simulink model "dev_switch_ekf"  (Simulink 7.0)
settings: Solver=FixedStepDiscrete  StartTime=0  StopTime=100  FixedStep=1e-3  RelTol=1e-3
undefined symbols (not defined in the file): l_fts, Q_in, R_n9, ts, zmsr
libraries: simulink x14, DLRwalkerLib x3, DLRHumanoid x2
(part 1 of 2)
settings Model: Creator=raje_ra  LastModifiedBy=raje_ra  ExtModeAutoUpdateStatusClock=off

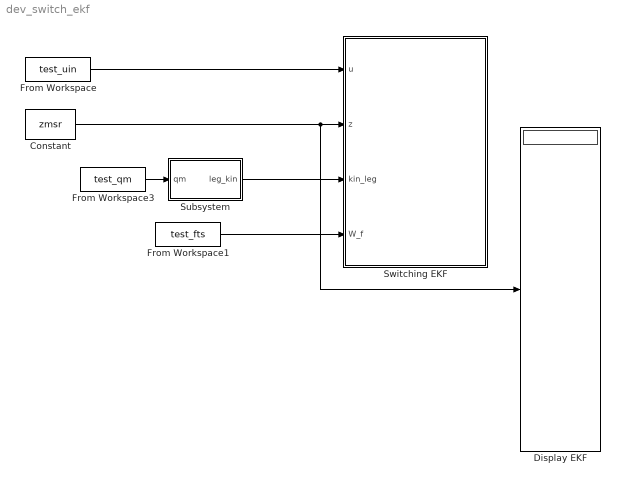
== system dev_switch_ekf ==
  Constant : Constant  Value=zmsr  OutDataType=sfix(16)  OutScaling=2^0
  Display EKF : Display
  From Workspace : FromWorkspace  VariableName=test_uin  SampleTime=0  OutputAfterFinalValue=Setting to zero
  From Workspace1 : FromWorkspace  VariableName=test_fts  SampleTime=0  OutputAfterFinalValue=Setting to zero
  From Workspace3 : FromWorkspace  VariableName=test_qm  SampleTime=0  OutputAfterFinalValue=Setting to zero
  Subsystem : Subsystem
  Switching EKF : Subsystem
  wires:
  From Workspace3/1 -> Subsystem/1(qm)
  Subsystem/1(leg_kin) -> Switching EKF/3(kin_leg)
  From Workspace1/1 -> Switching EKF/4(W_f)
  From Workspace/1 -> Switching EKF/1(u)
  Constant/1 -> Switching EKF/2(z), Display EKF/1

== system dev_switch_ekf/Subsystem ==
  qm : Inport  OutDataType=sfix(16)  OutScaling=2^0
  Bus Creator : BusCreator
  Fkin_leg_l : DLRHumanoid/Fkin_leg_l  SystemSampleTime=-1
  Fkin_leg_r : DLRHumanoid/Fkin_leg_r  SystemSampleTime=-1
  J_leg_l : Subsystem  AncestorBlock=DLRHumanoid/J_leg_l
  J_leg_r : Subsystem  AncestorBlock=DLRHumanoid/J_leg_r
  leg_kin : Outport  OutDataType=sfix(16)  OutScaling=2^0
  wires:
  qm/1 -> Fkin_leg_r/1, Fkin_leg_l/1, J_leg_r/1(q), J_leg_l/1(q)
  Fkin_leg_r/1 -> Bus Creator/1  "Fkin_leg_r"
  Bus Creator/1 -> leg_kin/1
  Fkin_leg_l/1 -> Bus Creator/2  "Fkin_leg_l"
  J_leg_r/1(J) -> Bus Creator/3  "J_leg_r"
  J_leg_l/1(J) -> Bus Creator/4  "J_leg_l"

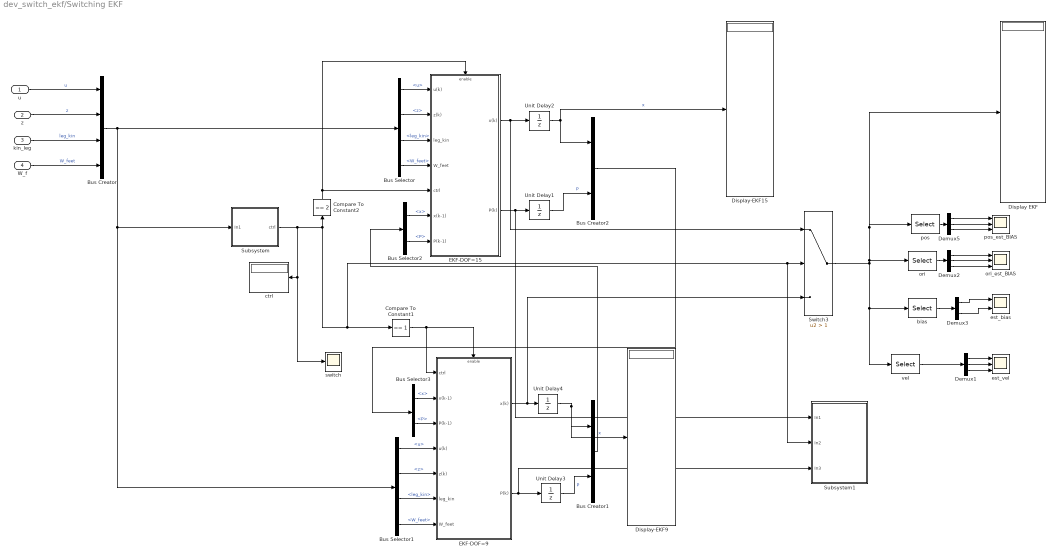
== system dev_switch_ekf/Switching EKF ==
  u : Inport
  z : Inport  Port=2
  kin_leg : Inport  Port=3
  W_f : Inport  Port=4
  Bus Creator : BusCreator
  Bus Creator1 : BusCreator  Inputs=2
  Bus Creator2 : BusCreator  Inputs=2
  Bus Selector : BusSelector  OutputSignals=u,z,leg_kin,W_feet
  Bus Selector1 : BusSelector  OutputSignals=u,z,leg_kin,W_feet
  Bus Selector2 : BusSelector  OutputSignals=x,P
  Bus Selector3 : BusSelector  OutputSignals=x,P
  Compare To Constant1 : simulink/Logic and Bit Operations/Compare To Constant  SystemSampleTime=-1  relop===  const=1  LogicOutDataTypeMode=uint8  ZeroCross=off
  Compare To Constant2 : simulink/Logic and Bit Operations/Compare To Constant  Orientation=up  SystemSampleTime=-1  relop===  const=2  LogicOutDataTypeMode=uint8  ZeroCross=off
  Demux1 : Demux  Outputs=3
  Demux2 : Demux  Outputs=3
  Demux3 : Demux  Outputs=2
  Demux5 : Demux  Outputs=3
  Display EKF : Display
  Display-EKF15 : Display
  Display-EKF9 : Display
  EKF-DOF=15 : Subsystem
  EKF-DOF=9 : Subsystem
  Subsystem : Subsystem
  Subsystem1 : Subsystem
  Switch3 : Switch  Criteria=u2 > Threshold  Threshold=1  OutDataType=sfix(16)  OutScaling=2^0
  Unit Delay1 : UnitDelay  X0=zeros(15)  SampleTime=-1
  Unit Delay2 : UnitDelay  X0=zeros(15,1)  SampleTime=-1
  Unit Delay3 : UnitDelay  X0=eye(15)  SampleTime=-1
  Unit Delay4 : UnitDelay  X0=zeros(15,1)  SampleTime=-1
  bias : Selector  InputPortWidth=15  IndexOptions=Index vector (dialog)  Indices=10:15  OutputSizes=1
  ctrl : Display
      settings: Decimation=100
  est_bias : Scope  NumInputPorts=2
      settings: TickLabels=on  TimeRange=10  YMin=-0.08~-0.14  YMax=0.14~0.06  SaveName=ScopeData117
  est_vel : Scope  NumInputPorts=3
      settings: TickLabels=on  TimeRange=1  YMin=-0.025~-8.67362e-19~-0.02  YMax=0.0025~0.04~0.002
  ori : Selector  InputPortWidth=15  IndexOptions=Index vector (dialog)  Indices=4:6  OutputSizes=1
  ori_est_BIAS : Scope  NumInputPorts=3
      settings: TickLabels=on  TimeRange=10  YMin=-0.009000000000000001~-0.12~-0.026  YMax=-0.003000000000000001~0.04000000000000001~-0.012  SaveName=ScopeData109
  pos : Selector  InputPortWidth=15  IndexOptions=Index vector (dialog)  Indices=1:3  OutputSizes=1
  pos_est_BIAS : Scope  NumInputPorts=3
      settings: TickLabels=on  TimeRange=30  YMin=-0.004~-0.025~1.161  YMax=0.0055~0.275~1.175  SaveName=ScopeData128
  switch : Scope
      settings: TickLabels=on  TimeRange=1  YMin=-0.025  YMax=0.0025  SaveName=ScopeData4
  vel : Selector  InputPortWidth=15  IndexOptions=Index vector (dialog)  Indices=7:9  OutputSizes=1
  wires:
  ori/1 -> Demux2/1
  Demux2/1 -> ori_est_BIAS/1
  Demux2/2 -> ori_est_BIAS/2
  Demux2/3 -> ori_est_BIAS/3
  bias/1 -> Demux3/1
  Demux3/1 -> est_bias/1
  Demux3/2 -> est_bias/2
  pos/1 -> Demux5/1
  Demux5/1 -> pos_est_BIAS/1
  Demux5/2 -> pos_est_BIAS/2
  Demux5/3 -> pos_est_BIAS/3
  u/1 -> Bus Creator/1  "u"
  z/1 -> Bus Creator/2  "z"
  kin_leg/1 -> Bus Creator/3  "leg_kin"
  W_f/1 -> Bus Creator/4  "W_feet"
  Bus Creator/1 -> Bus Selector/1, Bus Selector1/1, Subsystem/1(In1)
  Bus Selector/1 -> EKF-DOF=15/1(u(k))  "<u>"
  Bus Selector/2 -> EKF-DOF=15/2(z(k))  "<z>"
  Bus Selector/3 -> EKF-DOF=15/3(leg_kin)  "<leg_kin>"
  Bus Selector/4 -> EKF-DOF=15/4(W_feet)  "<W_feet>"
  Bus Selector1/1 -> EKF-DOF=9/4(u(k))  "<u>"
  Bus Selector1/2 -> EKF-DOF=9/5(z(k))  "<z>"
  Bus Selector1/3 -> EKF-DOF=9/6(leg_kin)  "<leg_kin>"
  Bus Selector1/4 -> EKF-DOF=9/7(W_feet)  "<W_feet>"
  EKF-DOF=15/1(x(k)) -> Unit Delay2/1, Switch3/1
  EKF-DOF=15/2(P(k)) -> Unit Delay1/1, Subsystem1/1(In1)
  Compare To Constant1/1 -> EKF-DOF=9/1(ctrl), EKF-DOF=9/Enable
  Subsystem/1(ctrl) -> Compare To Constant1/1, Switch3/2, Subsystem1/2(In2), Compare To Constant2/1, ctrl/1, switch/1
  EKF-DOF=9/1(x(k)) -> Unit Delay4/1, Switch3/3
  EKF-DOF=9/2(P(k)) -> Unit Delay3/1, Subsystem1/3(In3)
  Unit Delay4/1 -> Bus Creator1/1, Display-EKF9/1  "x"
  Unit Delay3/1 -> Bus Creator1/2  "P"
  Unit Delay2/1 -> Bus Creator2/1, Display-EKF15/1  "x"
  Unit Delay1/1 -> Bus Creator2/2  "P"
  Bus Selector2/1 -> EKF-DOF=15/6(x(k-1))  "<x>"
  Bus Selector2/2 -> EKF-DOF=15/7(P(k-1))  "<P>"
  Bus Selector3/1 -> EKF-DOF=9/2(x(k-1))  "<x>"
  Bus Selector3/2 -> EKF-DOF=9/3(P(k-1))  "<P>"
  Bus Creator2/1 -> Bus Selector3/1
  Bus Creator1/1 -> Bus Selector2/1
  Switch3/1 -> ori/1, pos/1, Display EKF/1, bias/1, vel/1
  Compare To Constant2/1 -> EKF-DOF=15/5(ctrl), EKF-DOF=15/Enable
  Demux1/1 -> est_vel/1
  Demux1/2 -> est_vel/2
  Demux1/3 -> est_vel/3
  vel/1 -> Demux1/1

== system dev_switch_ekf/Subsystem/J_leg_l ==
  q : Inport
  Reshape10 : Reshape  OutputDimensionality=Customize  OutputDimensions=[6,6]
  S-Function1 : S-Function  FunctionName=sJ_leg_l  Parameters=kinpar
  J : Outport
  wires:
  q/1 -> S-Function1/1
  Reshape10/1 -> J/1
  S-Function1/1 -> Reshape10/1

== system dev_switch_ekf/Subsystem/J_leg_r ==
  q : Inport
  Reshape10 : Reshape  OutputDimensionality=Customize  OutputDimensions=[6,6]
  S-Function4 : S-Function  FunctionName=sJ_leg_r  Parameters=kinpar
  J : Outport
  wires:
  S-Function4/1 -> Reshape10/1
  Reshape10/1 -> J/1
  q/1 -> S-Function4/1

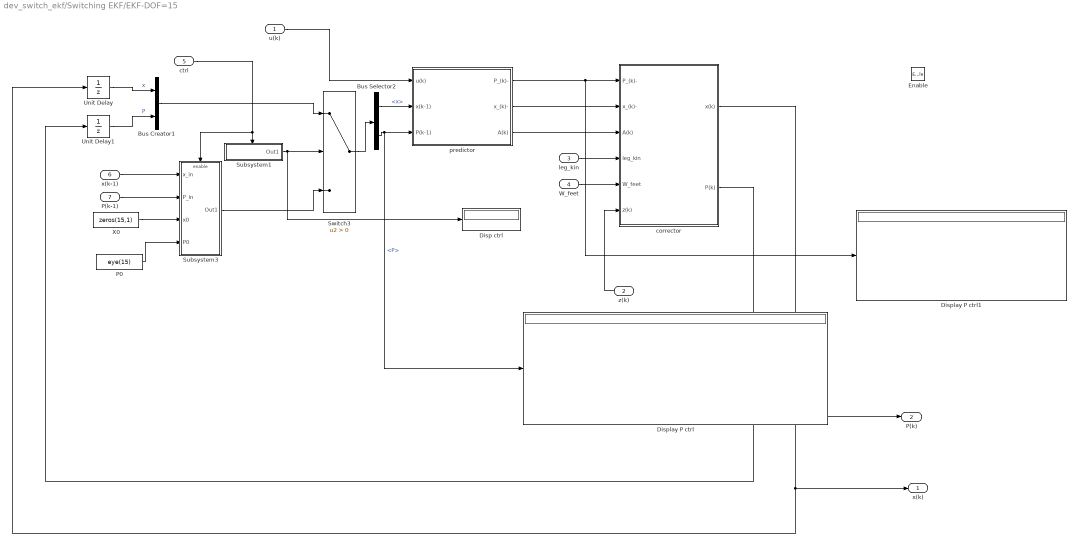
== system dev_switch_ekf/Switching EKF/EKF-DOF=15 ==
  u(k) : Inport  OutDataType=sfix(16)  OutScaling=2^0
  z(k) : Inport  Orientation=left  Port=2  OutDataType=sfix(16)  OutScaling=2^0
  leg_kin : Inport  Port=3  OutDataType=sfix(16)  OutScaling=2^0
  W_feet : Inport  Port=4  OutDataType=sfix(16)  OutScaling=2^0
  ctrl : Inport  Port=5  OutDataType=sfix(16)  OutScaling=2^0
  x(k-1) : Inport  Port=6  OutDataType=sfix(16)  OutScaling=2^0
  P(k-1) : Inport  Port=7  OutDataType=sfix(16)  OutScaling=2^0
  Enable : EnablePort  StatesWhenEnabling=reset
  Bus Creator1 : BusCreator  Inputs=2
  Bus Selector2 : BusSelector  OutputSignals=x,P
  Disp ctrl : Display
  Display P ctrl : Display
  Display P ctrl1 : Display
  P0 : Constant  Value=eye(15)  VectorParams1D=off  OutDataType=sfix(16)  OutScaling=2^0
  Subsystem1 : Subsystem
  Subsystem3 : Subsystem
  Switch3 : Switch  Criteria=u2 > Threshold  OutDataType=sfix(16)  OutScaling=2^0
  Unit Delay : UnitDelay  X0=zeros(15,1)  SampleTime=ts
  Unit Delay1 : UnitDelay  X0=zeros(15)  SampleTime=ts
  X0 : Constant  Value=zeros(15,1)  OutDataType=sfix(16)  OutScaling=2^0
  corrector : Subsystem
  predictor : Subsystem
  x(k) : Outport  OutDataType=sfix(16)  OutScaling=2^0
  P(k) : Outport  Port=2  OutDataType=sfix(16)  OutScaling=2^0
  wires:
  corrector/2(P(k)) -> Unit Delay1/1, P(k)/1
  predictor/1(P_(k)-) -> corrector/1(P_(k)-), Display P ctrl1/1
  corrector/1(x(k)) -> Unit Delay/1, x(k)/1
  predictor/2(x_(k)-) -> corrector/2(x_(k)-)
  u(k)/1 -> predictor/1(u(k))
  leg_kin/1 -> corrector/4(leg_kin)
  W_feet/1 -> corrector/5(W_feet)
  z(k)/1 -> corrector/6(z(k))
  predictor/3(A(k)) -> corrector/3(A(k))
  Subsystem1/1(Out1) -> Switch3/2, Disp ctrl/1
  ctrl/1 -> Subsystem1/Enable, Subsystem3/Enable
  Subsystem3/1(Out1) -> Switch3/3
  X0/1 -> Subsystem3/3(x0)
  P0/1 -> Subsystem3/4(P0)
  x(k-1)/1 -> Subsystem3/1(x_in)
  P(k-1)/1 -> Subsystem3/2(P_in)
  Unit Delay/1 -> Bus Creator1/1  "x"
  Unit Delay1/1 -> Bus Creator1/2  "P"
  Bus Creator1/1 -> Switch3/1
  Switch3/1 -> Bus Selector2/1
  Bus Selector2/1 -> predictor/2(x(k-1))  "<x>"
  Bus Selector2/2 -> predictor/3(P(k-1)), Display P ctrl/1  "<P>"

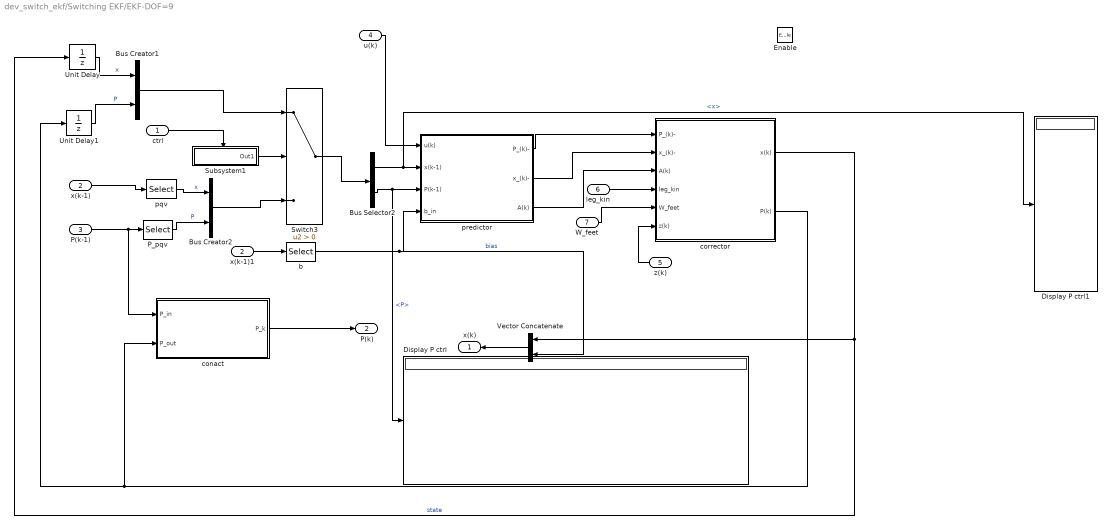
== system dev_switch_ekf/Switching EKF/EKF-DOF=9 ==
  ctrl : Inport  OutDataType=sfix(16)  OutScaling=2^0
  x(k-1) : Inport  Port=2  OutDataType=sfix(16)  OutScaling=2^0
  P(k-1) : Inport  Port=3  OutDataType=sfix(16)  OutScaling=2^0
  u(k) : Inport  Port=4  OutDataType=sfix(16)  OutScaling=2^0
  z(k) : Inport  Orientation=left  Port=5  OutDataType=sfix(16)  OutScaling=2^0
  leg_kin : Inport  Port=6  OutDataType=sfix(16)  OutScaling=2^0
  W_feet : Inport  Port=7  OutDataType=sfix(16)  OutScaling=2^0
  Enable : EnablePort  StatesWhenEnabling=reset
  Bus Creator1 : BusCreator  Inputs=2
  Bus Creator2 : BusCreator  Inputs=2
  Bus Selector2 : BusSelector  OutputSignals=x,P
  Display P ctrl : Display
  Display P ctrl1 : Display
  P_pqv : Selector  NumberOfDimensions=2  InputPortWidth=15  IndexOptions=Index vector (dialog),Index vector (dialog)  Indices=1:9,1:9  OutputSizes=1,1
  Subsystem1 : Subsystem
  Switch3 : Switch  Criteria=u2 > Threshold  OutDataType=sfix(16)  OutScaling=2^0
  Unit Delay : UnitDelay  X0=zeros(9,1)  SampleTime=ts
  Unit Delay1 : UnitDelay  X0=eye(9)  SampleTime=ts
  Vector Concatenate : Concatenate  Orientation=left  Mode=Vector
  b : Selector  InputPortWidth=15  IndexOptions=Index vector (dialog)  Indices=10:15  OutputSizes=1
  conact : Stateflow chart
  corrector : Subsystem
  pqv : Selector  InputPortWidth=15  IndexOptions=Index vector (dialog)  Indices=1:9  OutputSizes=1
  predictor : Subsystem
  x(k-1)1 : InportShadow  Port=2  OutDataType=sfix(16)  OutScaling=2^0  LatchByCopyingInsideSignal=off
  x(k) : Outport  Orientation=left  OutDataType=sfix(16)  OutScaling=2^0
  P(k) : Outport  Port=2  OutDataType=sfix(16)  OutScaling=2^0
  wires:
  predictor/3(A(k)) -> corrector/3(A(k))
  z(k)/1 -> corrector/6(z(k))
  W_feet/1 -> corrector/5(W_feet)
  leg_kin/1 -> corrector/4(leg_kin)
  u(k)/1 -> predictor/1(u(k))
  predictor/2(x_(k)-) -> corrector/2(x_(k)-)
  corrector/1(x(k)) -> Vector Concatenate/1, Unit Delay/1  "state"
  predictor/1(P_(k)-) -> corrector/1(P_(k)-)
  corrector/2(P(k)) -> Unit Delay1/1, conact/2(P_out)
  Subsystem1/1(Out1) -> Switch3/2
  x(k-1)/1 -> pqv/1
  ctrl/1 -> Subsystem1/Enable
  P(k-1)/1 -> P_pqv/1, conact/1(P_in)
  b/1 -> predictor/4(b_in), Vector Concatenate/2  "bias"
  Vector Concatenate/1 -> x(k)/1
  conact/1(P_k) -> P(k)/1
  Unit Delay/1 -> Bus Creator1/1  "x"
  Unit Delay1/1 -> Bus Creator1/2  "P"
  Bus Creator1/1 -> Switch3/1
  P_pqv/1 -> Bus Creator2/2  "P"
  pqv/1 -> Bus Creator2/1  "x"
  Bus Creator2/1 -> Switch3/3
  Switch3/1 -> Bus Selector2/1
  Bus Selector2/1 -> predictor/2(x(k-1)), Display P ctrl1/1  "<x>"
  Bus Selector2/2 -> predictor/3(P(k-1)), Display P ctrl/1  "<P>"
  x(k-1)1/1 -> b/1

== system dev_switch_ekf/Switching EKF/Subsystem ==
  note: 1..single left leg
      | 2.. single right leg
      | 3.. double support
      | 4.. flying
  In1 : Inport
  Bus Selector2 : BusSelector  OutputSignals=W_feet
  Demux : Demux  Outputs=2
  ZMP Calculator : Subsystem
  conact : Stateflow chart
  ctrl : Outport
  wires:
  Bus Selector2/1 -> Demux/1  "<W_feet>"
  Demux/2 -> ZMP Calculator/2(WL)
  Demux/1 -> ZMP Calculator/1(WR)
  ZMP Calculator/1(pcalc) -> conact/1(zmp)
  ZMP Calculator/2(cnt_state) -> conact/2(state)
  In1/1 -> Bus Selector2/1
  conact/1(y) -> ctrl/1

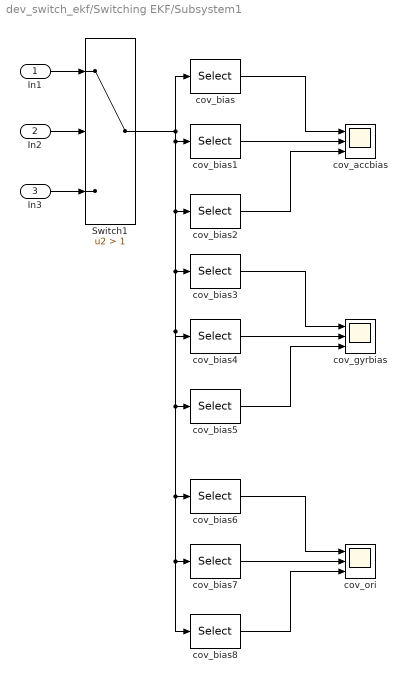
== system dev_switch_ekf/Switching EKF/Subsystem1 ==
  In1 : Inport
  In2 : Inport  Port=2
  In3 : Inport  Port=3
  Switch1 : Switch  Criteria=u2 > Threshold  Threshold=1  OutDataType=sfix(16)  OutScaling=2^0
  cov_accbias : Scope  NumInputPorts=3
      settings: TickLabels=on  TimeRange=1  YMin=-0.025~-8.67362e-19~-0.02  YMax=0.0025~0.04~0.002
  cov_bias : Selector  NumberOfDimensions=2  InputPortWidth=15  IndexOptions=Index vector (dialog),Index vector (dialog)  Indices=10,10  OutputSizes=1,1
  cov_bias1 : Selector  NumberOfDimensions=2  InputPortWidth=15  IndexOptions=Index vector (dialog),Index vector (dialog)  Indices=11,11  OutputSizes=1,1
  cov_bias2 : Selector  NumberOfDimensions=2  InputPortWidth=15  IndexOptions=Index vector (dialog),Index vector (dialog)  Indices=12,12  OutputSizes=1,1
  cov_bias3 : Selector  NumberOfDimensions=2  InputPortWidth=15  IndexOptions=Index vector (dialog),Index vector (dialog)  Indices=13,13  OutputSizes=1,1
  cov_bias4 : Selector  NumberOfDimensions=2  InputPortWidth=15  IndexOptions=Index vector (dialog),Index vector (dialog)  Indices=14,14  OutputSizes=1,1
  cov_bias5 : Selector  NumberOfDimensions=2  InputPortWidth=15  IndexOptions=Index vector (dialog),Index vector (dialog)  Indices=15,15  OutputSizes=1,1
  cov_bias6 : Selector  NumberOfDimensions=2  InputPortWidth=15  IndexOptions=Index vector (dialog),Index vector (dialog)  Indices=4,4  OutputSizes=1,1
  cov_bias7 : Selector  NumberOfDimensions=2  InputPortWidth=15  IndexOptions=Index vector (dialog),Index vector (dialog)  Indices=5,5  OutputSizes=1,1
  cov_bias8 : Selector  NumberOfDimensions=2  InputPortWidth=15  IndexOptions=Index vector (dialog),Index vector (dialog)  Indices=6,6  OutputSizes=1,1
  cov_gyrbias : Scope  NumInputPorts=3
      settings: TickLabels=on  TimeRange=1  YMin=-0.025~-8.67362e-19~-0.02  YMax=0.0025~0.04~0.002  SaveName=ScopeData2
  cov_ori : Scope  NumInputPorts=3
      settings: TickLabels=on  TimeRange=10  YMin=4e-12~0~4e-12  YMax=1.4e-11~7.000000000000001e-09~1.8e-11  SaveName=ScopeData3
  wires:
  Switch1/1 -> cov_bias/1, cov_bias1/1, cov_bias2/1, cov_bias3/1, cov_bias4/1, cov_bias5/1, cov_bias6/1, cov_bias7/1, cov_bias8/1
  cov_bias/1 -> cov_accbias/1
  cov_bias1/1 -> cov_accbias/2
  cov_bias2/1 -> cov_accbias/3
  cov_bias3/1 -> cov_gyrbias/1
  cov_bias4/1 -> cov_gyrbias/2
  cov_bias5/1 -> cov_gyrbias/3
  In1/1 -> Switch1/1
  In2/1 -> Switch1/2
  In3/1 -> Switch1/3
  cov_bias6/1 -> cov_ori/1
  cov_bias7/1 -> cov_ori/2
  cov_bias8/1 -> cov_ori/3

== system dev_switch_ekf/Switching EKF/EKF-DOF=15/Subsystem1 ==
  Enable : EnablePort  StatesWhenEnabling=reset
  Init/Run  Logik : DLRwalkerLib/Misc/Init//Run  Logik  SystemSampleTime=-1
  Terminator : Terminator
  Out1 : Outport
  wires:
  Init/Run  Logik/1 -> Terminator/1
  Init/Run  Logik/2 -> Out1/1

== system dev_switch_ekf/Switching EKF/EKF-DOF=15/Subsystem3 ==
  x_in : Inport  OutDataType=sfix(16)  OutScaling=2^0
  P_in : Inport  Port=2  OutDataType=sfix(16)  OutScaling=2^0
  x0 : Inport  Port=3  OutDataType=sfix(16)  OutScaling=2^0
  P0 : Inport  Port=4  OutDataType=sfix(16)  OutScaling=2^0
  Enable : EnablePort  ShowOutputPort=on
  Bus Creator1 : BusCreator  Inputs=2
  Bus Creator2 : BusCreator  Inputs=2
  Init/Run  Logik : DLRwalkerLib/Misc/Init//Run  Logik  SystemSampleTime=-1
  Switch : Switch  Criteria=u2 > Threshold  OutDataType=sfix(16)  OutScaling=2^0
  Terminator : Terminator
  Out1 : Outport
  wires:
  Init/Run  Logik/2 -> Switch/2
  Init/Run  Logik/1 -> Terminator/1
  Switch/1 -> Out1/1
  x0/1 -> Bus Creator1/1  "x"
  P0/1 -> Bus Creator1/2  "P"
  Bus Creator1/1 -> Switch/3
  x_in/1 -> Bus Creator2/1  "x"
  P_in/1 -> Bus Creator2/2  "P"
  Bus Creator2/1 -> Switch/1

== system dev_switch_ekf/Switching EKF/EKF-DOF=15/corrector ==
  P_(k)- : Inport  OutDataType=sfix(16)  OutScaling=2^0
  x_(k)- : Inport  Port=2  OutDataType=sfix(16)  OutScaling=2^0
  A(k) : Inport  Port=3  OutDataType=sfix(16)  OutScaling=2^0
  leg_kin : Inport  Port=4  OutDataType=sfix(16)  OutScaling=2^0
  W_feet : Inport  Port=5  OutDataType=sfix(16)  OutScaling=2^0
  z(k) : Inport  Port=6  OutDataType=sfix(16)  OutScaling=2^0
  Bus Selector3 : BusSelector  OutputSignals=Fkin_leg_r,Fkin_leg_l
  Constant : Constant  Value=R_n9  OutDataType=sfix(16)  OutScaling=2^0
  Demux : Demux  Outputs=2
  Eul Rotation : Stateflow chart
  Measurement update1 : Stateflow chart
  Selector1 : Selector  InputPortWidth=15  IndexOptions=Index vector (dialog)  Indices=[1:6]  OutputSizes=1
  ZMP Calculator : Subsystem
  x(k) : Outport  OutDataType=sfix(16)  OutScaling=2^0
  P(k) : Outport  Port=2  OutDataType=sfix(16)  OutScaling=2^0
  wires:
  Measurement update1/1(x_k) -> x(k)/1
  x_(k)-/1 -> Measurement update1/1(x_in), Selector1/1
  Selector1/1 -> Eul Rotation/1(o)
  Eul Rotation/1(g) -> Measurement update1/3(g_in)
  Eul Rotation/2(dg) -> Measurement update1/4(dg_in)
  leg_kin/1 -> Bus Selector3/1
  Bus Selector3/1 -> Measurement update1/5(kin_rf)  "<Fkin_leg_r>"
  Bus Selector3/2 -> Measurement update1/6(kin_lf)  "<Fkin_leg_l>"
  Demux/1 -> ZMP Calculator/2(WR)
  Demux/2 -> ZMP Calculator/1(WL)
  W_feet/1 -> Demux/1
  ZMP Calculator/1(pcalc) -> Measurement update1/7(cnt_msr)
  ZMP Calculator/2(cnt_state) -> Measurement update1/8(state)
  P_(k)-/1 -> Measurement update1/10(P_)
  Constant/1 -> Measurement update1/9(R_in)
  Measurement update1/2(P) -> P(k)/1  "H"
  z(k)/1 -> Measurement update1/11(z)
  A(k)/1 -> Measurement update1/2(A)

== system dev_switch_ekf/Switching EKF/EKF-DOF=15/predictor ==
  u(k) : Inport  OutDataType=sfix(16)  OutScaling=2^0
  x(k-1) : Inport  Port=2  OutDataType=sfix(16)  OutScaling=2^0
  P(k-1) : Inport  Port=3  OutDataType=sfix(16)  OutScaling=2^0
  Analytical Jacobian1 : Stateflow chart
  Constant2 : Constant  Value=Q_in  VectorParams1D=off  OutDataType=sfix(16)  OutScaling=2^0
  Display P ctrl1 : Display
  Eul Rotation1 : Stateflow chart
  Math Function : Math  Operator=transpose  OutDataType=sfix(16)  OutScaling=2^0  SaturateOnIntegerOverflow=on
  Process noise : Stateflow chart
  Product : Product  Inputs=3  Multiplication=Matrix(*)  OutDataType=sfix(16)  OutScaling=2^0  RndMeth=Zero
  Selector : Selector  InputPortWidth=15  IndexOptions=Index vector (dialog)  Indices=[4 5 6]  OutputSizes=1
  Sum1 : Sum  Inputs=|++  OutDataType=sfix(16)  OutScaling=2^0
  Time Update : Stateflow chart
  P_(k)- : Outport  OutDataType=sfix(16)  OutScaling=2^0
  x_(k)- : Outport  Port=2  OutDataType=sfix(16)  OutScaling=2^0
  A(k) : Outport  Port=3  OutDataType=sfix(16)  OutScaling=2^0
  wires:
  Eul Rotation1/2(dR) -> Time Update/5(dR)
  Eul Rotation1/1(R) -> Time Update/4(R), Process noise/2(R)
  Analytical Jacobian1/2(dinvT) -> Time Update/3(dinvT)
  Analytical Jacobian1/1(invT) -> Time Update/2(invT), Process noise/1(invT)
  Selector/1 -> Analytical Jacobian1/1(o), Eul Rotation1/1(o)
  Time Update/2(x_k) -> x_(k)-/1
  u(k)/1 -> Time Update/6(u_in)
  Sum1/1 -> P_(k)-/1
  Product/1 -> Sum1/1
  P(k-1)/1 -> Product/2
  Math Function/1 -> Product/3
  Time Update/1(A) -> Product/1, Math Function/1, A(k)/1
  x(k-1)/1 -> Selector/1, Time Update/1(x_in)
  Process noise/1(Q_out) -> Sum1/2
  Constant2/1 -> Process noise/3(Q_in)

== system dev_switch_ekf/Switching EKF/EKF-DOF=9/Subsystem1 ==
  Enable : EnablePort  StatesWhenEnabling=reset
  Init/Run  Logik : DLRwalkerLib/Misc/Init//Run  Logik  SystemSampleTime=-1
  Terminator : Terminator
  Out1 : Outport
  wires:
  Init/Run  Logik/2 -> Out1/1
  Init/Run  Logik/1 -> Terminator/1

== system dev_switch_ekf/Switching EKF/EKF-DOF=9/corrector ==
  P_(k)- : Inport  OutDataType=sfix(16)  OutScaling=2^0
  x_(k)- : Inport  Port=2  OutDataType=sfix(16)  OutScaling=2^0
  A(k) : Inport  Port=3  OutDataType=sfix(16)  OutScaling=2^0
  leg_kin : Inport  Port=4  OutDataType=sfix(16)  OutScaling=2^0
  W_feet : Inport  Port=5  OutDataType=sfix(16)  OutScaling=2^0
  z(k) : Inport  Port=6  OutDataType=sfix(16)  OutScaling=2^0
  Bus Selector3 : BusSelector  OutputSignals=Fkin_leg_r,Fkin_leg_l
  Constant : Constant  Value=R_n9  OutDataType=sfix(16)  OutScaling=2^0
  Demux : Demux  Outputs=2
  Eul Rotation : Stateflow chart
  Measurement update1 : Stateflow chart
  Selector1 : Selector  InputPortWidth=9  IndexOptions=Index vector (dialog)  Indices=[1:6]  OutputSizes=1
  ZMP Calculator : Subsystem
  x(k) : Outport  OutDataType=sfix(16)  OutScaling=2^0
  P(k) : Outport  Port=2  OutDataType=sfix(16)  OutScaling=2^0
  wires:
  A(k)/1 -> Measurement update1/2(A)
  z(k)/1 -> Measurement update1/11(z)
  Measurement update1/2(P) -> P(k)/1  "H"
  Constant/1 -> Measurement update1/9(R_in)
  P_(k)-/1 -> Measurement update1/10(P_)
  ZMP Calculator/2(cnt_state) -> Measurement update1/8(state)
  ZMP Calculator/1(pcalc) -> Measurement update1/7(cnt_msr)
  W_feet/1 -> Demux/1
  Demux/2 -> ZMP Calculator/1(WL)
  Demux/1 -> ZMP Calculator/2(WR)
  Bus Selector3/2 -> Measurement update1/6(kin_lf)  "<Fkin_leg_l>"
  Bus Selector3/1 -> Measurement update1/5(kin_rf)  "<Fkin_leg_r>"
  leg_kin/1 -> Bus Selector3/1
  Eul Rotation/2(dg) -> Measurement update1/4(dg_in)
  Eul Rotation/1(g) -> Measurement update1/3(g_in)
  Selector1/1 -> Eul Rotation/1(o)
  x_(k)-/1 -> Selector1/1, Measurement update1/1(x_in)
  Measurement update1/1(x_k) -> x(k)/1

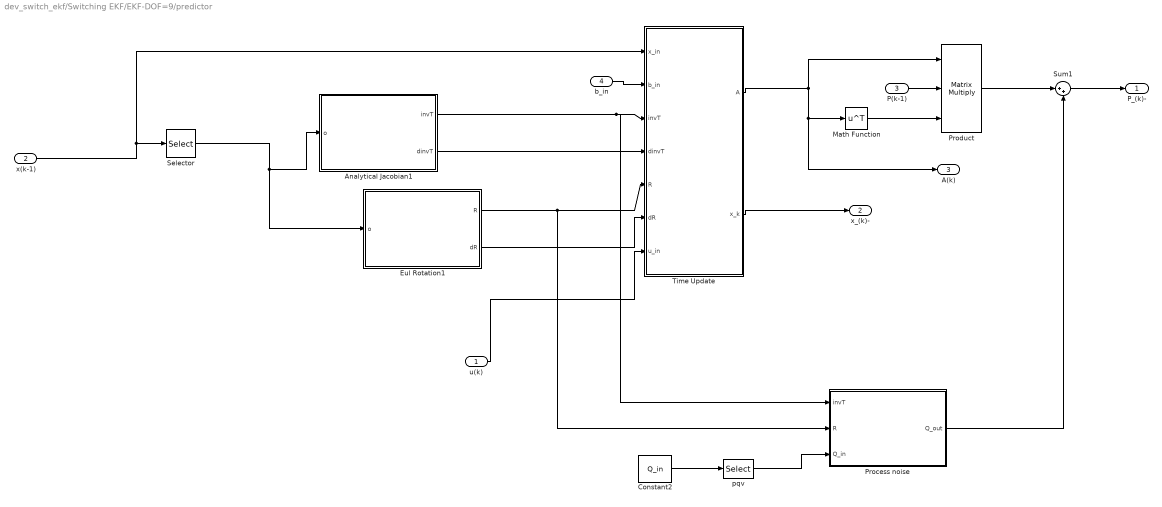
== system dev_switch_ekf/Switching EKF/EKF-DOF=9/predictor ==
  u(k) : Inport  OutDataType=sfix(16)  OutScaling=2^0
  x(k-1) : Inport  Port=2  OutDataType=sfix(16)  OutScaling=2^0
  P(k-1) : Inport  Port=3  OutDataType=sfix(16)  OutScaling=2^0
  b_in : Inport  Port=4  OutDataType=sfix(16)  OutScaling=2^0
  Analytical Jacobian1 : Stateflow chart
  Constant2 : Constant  Value=Q_in  VectorParams1D=off  OutDataType=sfix(16)  OutScaling=2^0
  Eul Rotation1 : Stateflow chart
  Math Function : Math  Operator=transpose  OutDataType=sfix(16)  OutScaling=2^0  SaturateOnIntegerOverflow=on
  Process noise : Stateflow chart
  Product : Product  Inputs=3  Multiplication=Matrix(*)  OutDataType=sfix(16)  OutScaling=2^0  RndMeth=Zero
  Selector : Selector  InputPortWidth=9  IndexOptions=Index vector (dialog)  Indices=[4 5 6]  OutputSizes=1
  Sum1 : Sum  Inputs=|++  OutDataType=sfix(16)  OutScaling=2^0
  Time Update : Stateflow chart
  pqv : Selector  NumberOfDimensions=2  InputPortWidth=15  IndexOptions=Index vector (dialog),Index vector (dialog)  Indices=1:6,1:6  OutputSizes=1,1
  P_(k)- : Outport  OutDataType=sfix(16)  OutScaling=2^0
  x_(k)- : Outport  Port=2  OutDataType=sfix(16)  OutScaling=2^0
  A(k) : Outport  Port=3  OutDataType=sfix(16)  OutScaling=2^0
  wires:
  x(k-1)/1 -> Time Update/1(x_in), Selector/1
  Time Update/1(A) -> A(k)/1, Math Function/1, Product/1
  Math Function/1 -> Product/3
  P(k-1)/1 -> Product/2
  Product/1 -> Sum1/1
  Sum1/1 -> P_(k)-/1
  u(k)/1 -> Time Update/7(u_in)
  Time Update/2(x_k) -> x_(k)-/1
  Selector/1 -> Eul Rotation1/1(o), Analytical Jacobian1/1(o)
  Analytical Jacobian1/1(invT) -> Time Update/3(invT), Process noise/1(invT)
  Analytical Jacobian1/2(dinvT) -> Time Update/4(dinvT)
  Eul Rotation1/1(R) -> Time Update/5(R), Process noise/2(R)
  Eul Rotation1/2(dR) -> Time Update/6(dR)
  b_in/1 -> Time Update/2(b_in)
  pqv/1 -> Process noise/3(Q_in)
  Constant2/1 -> pqv/1
  Process noise/1(Q_out) -> Sum1/2

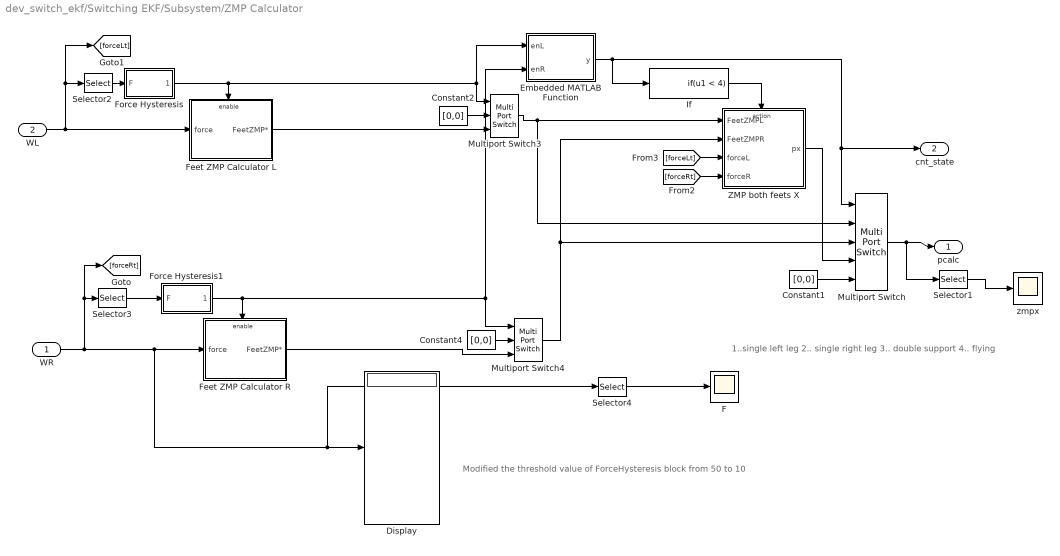
== system dev_switch_ekf/Switching EKF/Subsystem/ZMP Calculator ==
  note: Modified the threshold value of ForceHysteresis block from 50 to 10
  note: 1..single left leg
      | 2.. single right leg
      | 3.. double support
      | 4.. flying
  WR : Inport  OutDataType=sfix(16)  OutScaling=2^0
  WL : Inport  Port=2  OutDataType=sfix(16)  OutScaling=2^0
  Constant1 : Constant  Value=[0,0]  OutDataType=sfix(16)  OutScaling=2^0  SampleTime=-1
  Constant2 : Constant  Value=[0,0]  OutDataType=sfix(16)  OutScaling=2^0  SampleTime=-1
  Constant4 : Constant  Value=[0,0]  OutDataType=sfix(16)  OutScaling=2^0  SampleTime=-1
  Display : Display
  Embedded MATLAB Function : Stateflow chart
  F : Scope
      settings: TickLabels=on  TimeRange=30  YMin=-25  YMax=375  SaveName=ScopeData133
  Feet ZMP Calculator L : Subsystem  TreatAsAtomicUnit=on
  Feet ZMP Calculator R : Subsystem  TreatAsAtomicUnit=on
  Force Hysteresis : Subsystem  mask{f0=10, d=10}
      mask prompts: f0 "Threshold value"; d "Threshold hysteresis"
  Force Hysteresis1 : Subsystem  mask{f0=10, d=10}
      mask prompts: f0 "Threshold value"; d "Threshold hysteresis"
  If : If  IfExpression=u1 < 4  ShowElse=off
  Multiport Switch : MultiPortSwitch
  Multiport Switch3 : MultiPortSwitch  Inputs=2  zeroidx=on
  Multiport Switch4 : MultiPortSwitch  Inputs=2  zeroidx=on
  Selector1 : Selector  InputPortWidth=2  IndexOptions=Index vector (dialog)  Indices=1  OutputSizes=1
  Selector2 : Selector  InputPortWidth=6  IndexOptions=Index vector (dialog)  Indices=3  OutputSizes=1
  Selector3 : Selector  InputPortWidth=6  IndexOptions=Index vector (dialog)  Indices=3  OutputSizes=1
  Selector4 : Selector  InputPortWidth=6  IndexOptions=Index vector (dialog)  Indices=1:3  OutputSizes=1
  ZMP both feets X : Subsystem  TreatAsAtomicUnit=on
  zmpx : Scope
      settings: TickLabels=on  TimeRange=30  YMin=-0.55  YMax=0.5  SaveName=ScopeData131
  pcalc : Outport  OutDataType=sfix(16)  OutScaling=2^0
  cnt_state : Outport  Port=2  OutDataType=sfix(16)  OutScaling=2^0
  wires:
  Force Hysteresis1/1(contact) -> Feet ZMP Calculator R/Enable, Multiport Switch4/1, Embedded MATLAB Function/2(enR)
  Selector3/1 -> Force Hysteresis1/1(F)
  Multiport Switch4/1 -> ZMP both feets X/2(FeetZMPR), Multiport Switch/3
  Constant4/1 -> Multiport Switch4/2
  Constant2/1 -> Multiport Switch3/2
  Force Hysteresis/1(contact) -> Feet ZMP Calculator L/Enable, Multiport Switch3/1, Embedded MATLAB Function/1(enL)
  Selector2/1 -> Force Hysteresis/1(F)
  WL/1 -> Selector2/1, [forceLt], Feet ZMP Calculator L/1(force)
  WR/1 -> Selector3/1, [forceRt], Feet ZMP Calculator R/1(force), Display/1, Selector4/1
  [forceLt] -> ZMP both feets X/3(forceL)
  [forceRt] -> ZMP both feets X/4(forceR)
  Multiport Switch3/1 -> ZMP both feets X/1(FeetZMPL), Multiport Switch/2
  Multiport Switch/1 -> pcalc/1, Selector1/1
  Feet ZMP Calculator L/1(FeetZMP*) -> Multiport Switch3/3
  Feet ZMP Calculator R/1(FeetZMP*) -> Multiport Switch4/3
  Constant1/1 -> Multiport Switch/5
  ZMP both feets X/1(px) -> Multiport Switch/4
  Embedded MATLAB Function/1(y) -> cnt_state/1, Multiport Switch/1, If/1
  If/1 -> ZMP both feets X/Action
  Selector1/1 -> zmpx/1
  Selector4/1 -> F/1

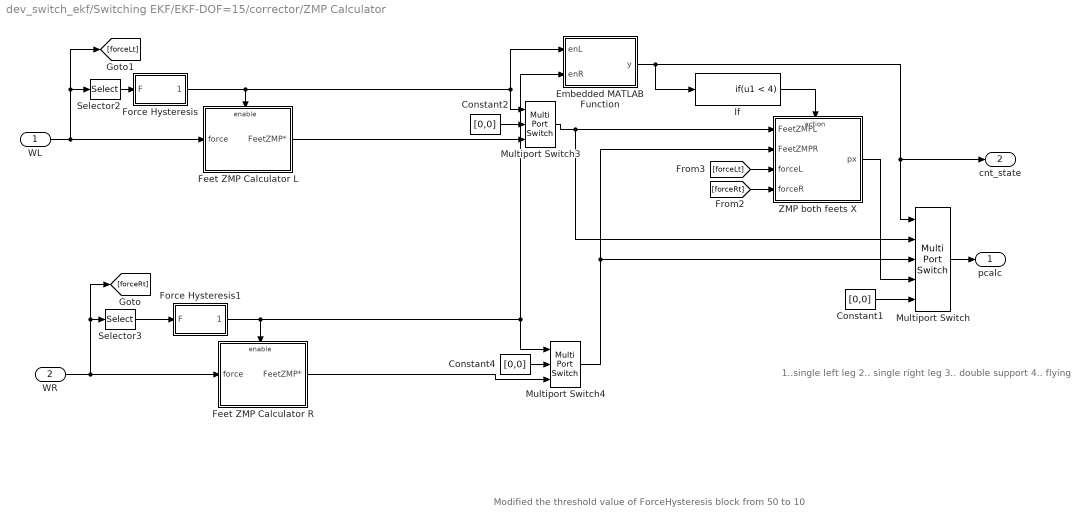
== system dev_switch_ekf/Switching EKF/EKF-DOF=15/corrector/ZMP Calculator ==
  note: 1..single left leg
      | 2.. single right leg
      | 3.. double support
      | 4.. flying
  note: Modified the threshold value of ForceHysteresis block from 50 to 10
  WL : Inport  OutDataType=sfix(16)  OutScaling=2^0
  WR : Inport  Port=2  OutDataType=sfix(16)  OutScaling=2^0
  Constant1 : Constant  Value=[0,0]  OutDataType=sfix(16)  OutScaling=2^0  SampleTime=-1
  Constant2 : Constant  Value=[0,0]  OutDataType=sfix(16)  OutScaling=2^0  SampleTime=-1
  Constant4 : Constant  Value=[0,0]  OutDataType=sfix(16)  OutScaling=2^0  SampleTime=-1
  Embedded MATLAB Function : Stateflow chart
  Feet ZMP Calculator L : Subsystem  TreatAsAtomicUnit=on
  Feet ZMP Calculator R : Subsystem  TreatAsAtomicUnit=on
  Force Hysteresis : Subsystem  mask{f0=10, d=10}
      mask prompts: f0 "Threshold value"; d "Threshold hysteresis"
  Force Hysteresis1 : Subsystem  mask{f0=10, d=10}
      mask prompts: f0 "Threshold value"; d "Threshold hysteresis"
  If : If  IfExpression=u1 < 4  ShowElse=off
  Multiport Switch : MultiPortSwitch
  Multiport Switch3 : MultiPortSwitch  Inputs=2  zeroidx=on
  Multiport Switch4 : MultiPortSwitch  Inputs=2  zeroidx=on
  Selector2 : Selector  InputPortWidth=6  IndexOptions=Index vector (dialog)  Indices=3  OutputSizes=1
  Selector3 : Selector  InputPortWidth=6  IndexOptions=Index vector (dialog)  Indices=3  OutputSizes=1
  ZMP both feets X : Subsystem  TreatAsAtomicUnit=on
  pcalc : Outport  OutDataType=sfix(16)  OutScaling=2^0
  cnt_state : Outport  Port=2  OutDataType=sfix(16)  OutScaling=2^0
  wires:
  If/1 -> ZMP both feets X/Action
  Embedded MATLAB Function/1(y) -> If/1, Multiport Switch/1, cnt_state/1
  ZMP both feets X/1(px) -> Multiport Switch/4
  Constant1/1 -> Multiport Switch/5
  Feet ZMP Calculator R/1(FeetZMP*) -> Multiport Switch4/3
  Feet ZMP Calculator L/1(FeetZMP*) -> Multiport Switch3/3
  Multiport Switch/1 -> pcalc/1
  Multiport Switch3/1 -> Multiport Switch/2, ZMP both feets X/1(FeetZMPL)
  [forceRt] -> ZMP both feets X/4(forceR)
  [forceLt] -> ZMP both feets X/3(forceL)
  WR/1 -> Feet ZMP Calculator R/1(force), [forceRt], Selector3/1
  WL/1 -> Feet ZMP Calculator L/1(force), [forceLt], Selector2/1
  Selector2/1 -> Force Hysteresis/1(F)
  Force Hysteresis/1(contact) -> Embedded MATLAB Function/1(enL), Multiport Switch3/1, Feet ZMP Calculator L/Enable
  Constant2/1 -> Multiport Switch3/2
  Constant4/1 -> Multiport Switch4/2
  Multiport Switch4/1 -> Multiport Switch/3, ZMP both feets X/2(FeetZMPR)
  Selector3/1 -> Force Hysteresis1/1(F)
  Force Hysteresis1/1(contact) -> Embedded MATLAB Function/2(enR), Multiport Switch4/1, Feet ZMP Calculator R/Enable

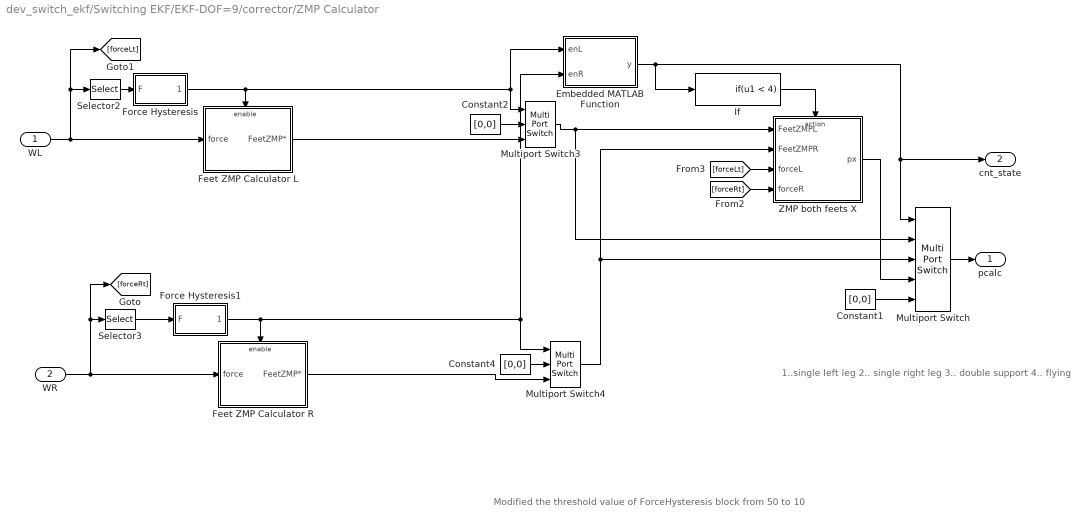
== system dev_switch_ekf/Switching EKF/EKF-DOF=9/corrector/ZMP Calculator ==
  note: Modified the threshold value of ForceHysteresis block from 50 to 10
  note: 1..single left leg
      | 2.. single right leg
      | 3.. double support
      | 4.. flying
  WL : Inport  OutDataType=sfix(16)  OutScaling=2^0
  WR : Inport  Port=2  OutDataType=sfix(16)  OutScaling=2^0
  Constant1 : Constant  Value=[0,0]  OutDataType=sfix(16)  OutScaling=2^0  SampleTime=-1
  Constant2 : Constant  Value=[0,0]  OutDataType=sfix(16)  OutScaling=2^0  SampleTime=-1
  Constant4 : Constant  Value=[0,0]  OutDataType=sfix(16)  OutScaling=2^0  SampleTime=-1
  Embedded MATLAB Function : Stateflow chart
  Feet ZMP Calculator L : Subsystem  TreatAsAtomicUnit=on
  Feet ZMP Calculator R : Subsystem  TreatAsAtomicUnit=on
  Force Hysteresis : Subsystem  mask{f0=10, d=10}
      mask prompts: f0 "Threshold value"; d "Threshold hysteresis"
  Force Hysteresis1 : Subsystem  mask{f0=10, d=10}
      mask prompts: f0 "Threshold value"; d "Threshold hysteresis"
  If : If  IfExpression=u1 < 4  ShowElse=off
  Multiport Switch : MultiPortSwitch
  Multiport Switch3 : MultiPortSwitch  Inputs=2  zeroidx=on
  Multiport Switch4 : MultiPortSwitch  Inputs=2  zeroidx=on
  Selector2 : Selector  InputPortWidth=6  IndexOptions=Index vector (dialog)  Indices=3  OutputSizes=1
  Selector3 : Selector  InputPortWidth=6  IndexOptions=Index vector (dialog)  Indices=3  OutputSizes=1
  ZMP both feets X : Subsystem  TreatAsAtomicUnit=on
  pcalc : Outport  OutDataType=sfix(16)  OutScaling=2^0
  cnt_state : Outport  Port=2  OutDataType=sfix(16)  OutScaling=2^0
  wires:
  Force Hysteresis1/1(contact) -> Feet ZMP Calculator R/Enable, Multiport Switch4/1, Embedded MATLAB Function/2(enR)
  Selector3/1 -> Force Hysteresis1/1(F)
  Multiport Switch4/1 -> ZMP both feets X/2(FeetZMPR), Multiport Switch/3
  Constant4/1 -> Multiport Switch4/2
  Constant2/1 -> Multiport Switch3/2
  Force Hysteresis/1(contact) -> Feet ZMP Calculator L/Enable, Multiport Switch3/1, Embedded MATLAB Function/1(enL)
  Selector2/1 -> Force Hysteresis/1(F)
  WL/1 -> Selector2/1, [forceLt], Feet ZMP Calculator L/1(force)
  WR/1 -> Selector3/1, [forceRt], Feet ZMP Calculator R/1(force)
  [forceLt] -> ZMP both feets X/3(forceL)
  [forceRt] -> ZMP both feets X/4(forceR)
  Multiport Switch3/1 -> ZMP both feets X/1(FeetZMPL), Multiport Switch/2
  Multiport Switch/1 -> pcalc/1
  Feet ZMP Calculator L/1(FeetZMP*) -> Multiport Switch3/3
  Feet ZMP Calculator R/1(FeetZMP*) -> Multiport Switch4/3
  Constant1/1 -> Multiport Switch/5
  ZMP both feets X/1(px) -> Multiport Switch/4
  Embedded MATLAB Function/1(y) -> cnt_state/1, Multiport Switch/1, If/1
  If/1 -> ZMP both feets X/Action

== system dev_switch_ekf/Switching EKF/Subsystem/ZMP Calculator/Feet ZMP Calculator L ==
  force : Inport  OutDataType=sfix(16)  OutScaling=2^0
  Enable : EnablePort  StatesWhenEnabling=reset
  Add : Sum  Inputs=--  OutDataType=sfix(16)  OutScaling=2^-10
  Add1 : Sum  Inputs=-+  OutDataType=sfix(16)  OutScaling=2^-10
  Demux : Demux  Outputs=6
  Divide : Product  Inputs=*/  OutDataType=sfix(16)  OutScaling=2^-10
  Divide1 : Product  Inputs=*/  OutDataType=sfix(16)  OutScaling=2^-10
  Gain : Gain  Gain=l_fts  ParameterDataType=sfix(16)  ParameterScaling=2^0  OutDataType=sfix(16)  OutScaling=2^0
  Gain1 : Gain  Gain=l_fts  ParameterDataType=sfix(16)  ParameterScaling=2^0  OutDataType=sfix(16)  OutScaling=2^0
  Mux1 : Mux  Inputs=2
  Terminator1 : Terminator
  FeetZMP* : Outport  OutDataType=sfix(16)  OutScaling=2^0
  wires:
  Mux1/1 -> FeetZMP*/1
  Gain/1 -> Add/1
  Demux/1 -> Gain/1
  Demux/5 -> Add/2
  Add/1 -> Divide/1
  force/1 -> Demux/1
  Gain1/1 -> Add1/1
  Add1/1 -> Divide1/1
  Demux/3 -> Divide/2, Divide1/2
  Demux/2 -> Gain1/1
  Demux/4 -> Add1/2
  Divide/1 -> Mux1/1
  Divide1/1 -> Mux1/2
  Demux/6 -> Terminator1/1

== system dev_switch_ekf/Switching EKF/Subsystem/ZMP Calculator/Feet ZMP Calculator R ==
  force : Inport  OutDataType=sfix(16)  OutScaling=2^0
  Enable : EnablePort  StatesWhenEnabling=reset
  Add : Sum  Inputs=--  OutDataType=sfix(16)  OutScaling=2^-10
  Add1 : Sum  Inputs=-+  OutDataType=sfix(16)  OutScaling=2^-10
  Demux : Demux  Outputs=6
  Divide : Product  Inputs=*/  OutDataType=sfix(16)  OutScaling=2^-10
  Divide1 : Product  Inputs=*/  OutDataType=sfix(16)  OutScaling=2^-10
  Gain : Gain  Gain=l_fts  ParameterDataType=sfix(16)  ParameterScaling=2^0  OutDataType=sfix(16)  OutScaling=2^0
  Gain1 : Gain  Gain=l_fts  ParameterDataType=sfix(16)  ParameterScaling=2^0  OutDataType=sfix(16)  OutScaling=2^0
  Mux1 : Mux  Inputs=2
  Terminator1 : Terminator
  FeetZMP* : Outport  OutDataType=sfix(16)  OutScaling=2^0
  wires:
  Divide1/1 -> Mux1/2
  Divide/1 -> Mux1/1
  Mux1/1 -> FeetZMP*/1
  Demux/4 -> Add1/2
  Demux/2 -> Gain1/1
  Demux/3 -> Divide1/2, Divide/2
  Add1/1 -> Divide1/1
  Gain1/1 -> Add1/1
  force/1 -> Demux/1
  Add/1 -> Divide/1
  Demux/5 -> Add/2
  Demux/1 -> Gain/1
  Gain/1 -> Add/1
  Demux/6 -> Terminator1/1

== system dev_switch_ekf/Switching EKF/Subsystem/ZMP Calculator/Force Hysteresis ==
  F : Inport
  Compare To Constant : simulink/Logic and Bit Operations/Compare To Constant  SystemSampleTime=-1  relop=<=  const=f0-d  LogicOutDataTypeMode=uint8  ZeroCross=off
  Compare To Constant1 : simulink/Logic and Bit Operations/Compare To Constant  SystemSampleTime=-1  relop=>=  const=f0+d  LogicOutDataTypeMode=uint8  ZeroCross=off
  Constant1 : Constant  OutDataType=sfix(16)  OutScaling=2^0
  Constant2 : Constant  Value=0  OutDataType=sfix(16)  OutScaling=2^0
  Switch : Switch  Threshold=0.5  OutDataType=sfix(16)  OutScaling=2^0
  Switch1 : Switch  Threshold=0.5  OutDataType=sfix(16)  OutScaling=2^0
  Unit Delay : UnitDelay  X0=1  SampleTime=ts
  contact : Outport  OutDataType=sfix(16)  OutScaling=2^0
  wires:
  Compare To Constant/1 -> Switch1/2
  Compare To Constant1/1 -> Switch/2
  Constant1/1 -> Switch/1
  Constant2/1 -> Switch1/1
  Switch1/1 -> Switch/3
  Unit Delay/1 -> Switch1/3
  Switch/1 -> Unit Delay/1, contact/1
  F/1 -> Compare To Constant/1, Compare To Constant1/1

== system dev_switch_ekf/Switching EKF/Subsystem/ZMP Calculator/Force Hysteresis1 ==
  F : Inport
  Compare To Constant : simulink/Logic and Bit Operations/Compare To Constant  SystemSampleTime=-1  relop=<=  const=f0-d  LogicOutDataTypeMode=uint8  ZeroCross=off
  Compare To Constant1 : simulink/Logic and Bit Operations/Compare To Constant  SystemSampleTime=-1  relop=>=  const=f0+d  LogicOutDataTypeMode=uint8  ZeroCross=off
  Constant1 : Constant  OutDataType=sfix(16)  OutScaling=2^0
  Constant2 : Constant  Value=0  OutDataType=sfix(16)  OutScaling=2^0
  Switch : Switch  Threshold=0.5  OutDataType=sfix(16)  OutScaling=2^0
  Switch1 : Switch  Threshold=0.5  OutDataType=sfix(16)  OutScaling=2^0
  Unit Delay : UnitDelay  X0=1  SampleTime=ts
  contact : Outport  OutDataType=sfix(16)  OutScaling=2^0
  wires:
  F/1 -> Compare To Constant1/1, Compare To Constant/1
  Switch/1 -> contact/1, Unit Delay/1
  Unit Delay/1 -> Switch1/3
  Switch1/1 -> Switch/3
  Constant2/1 -> Switch1/1
  Constant1/1 -> Switch/1
  Compare To Constant1/1 -> Switch/2
  Compare To Constant/1 -> Switch1/2

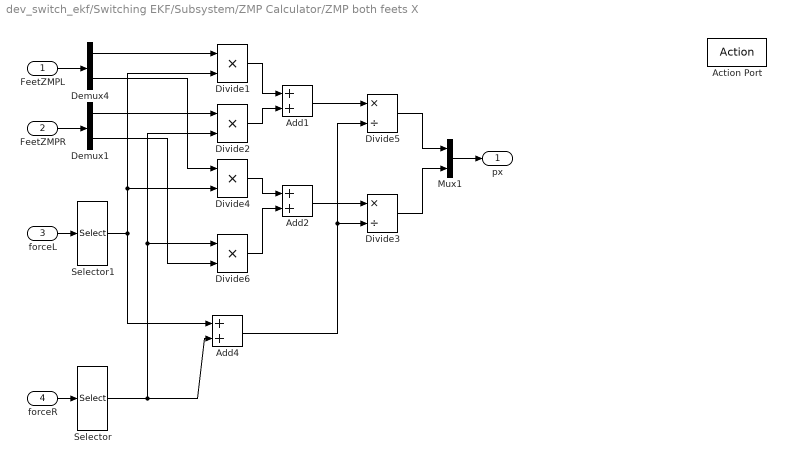
== system dev_switch_ekf/Switching EKF/Subsystem/ZMP Calculator/ZMP both feets X ==
  FeetZMPL : Inport  OutDataType=sfix(16)  OutScaling=2^0
  FeetZMPR : Inport  Port=2  OutDataType=sfix(16)  OutScaling=2^0
  forceL : Inport  Port=3  OutDataType=sfix(16)  OutScaling=2^0
  forceR : Inport  Port=4  OutDataType=sfix(16)  OutScaling=2^0
  Action Port : ActionPort  ActionType=then
  Add1 : Sum  OutDataType=sfix(16)  OutScaling=2^-10
  Add2 : Sum  OutDataType=sfix(16)  OutScaling=2^-10
  Add4 : Sum  OutDataType=sfix(16)  OutScaling=2^-10
  Demux1 : Demux  Outputs=2
  Demux4 : Demux  Outputs=2
  Divide{1..2,4,6} (4 alike) : Product  Inputs=**  OutDataType=sfix(16)  OutScaling=2^-10
  Divide3 : Product  Inputs=*/  OutDataType=sfix(16)  OutScaling=2^-10
  Divide5 : Product  Inputs=*/  OutDataType=sfix(16)  OutScaling=2^-10
  Mux1 : Mux  Inputs=2
  Selector : Selector  InputPortWidth=6  IndexOptions=Index vector (dialog)  Indices=[3]  OutputSizes=1
  Selector1 : Selector  InputPortWidth=6  IndexOptions=Index vector (dialog)  Indices=[3]  OutputSizes=1
  px : Outport  OutDataType=sfix(16)  OutScaling=2^0
  wires:
  forceR/1 -> Selector/1
  Selector/1 -> Add4/2, Divide2/2, Divide6/1
  Selector1/1 -> Add4/1, Divide1/2, Divide4/2
  forceL/1 -> Selector1/1
  Divide1/1 -> Add1/1
  Divide2/1 -> Add1/2
  Add1/1 -> Divide5/1
  Add4/1 -> Divide5/2, Divide3/2
  FeetZMPR/1 -> Demux1/1
  Demux1/1 -> Divide2/1
  FeetZMPL/1 -> Demux4/1
  Demux4/1 -> Divide1/1
  Divide4/1 -> Add2/1
  Divide6/1 -> Add2/2
  Demux4/2 -> Divide4/1
  Demux1/2 -> Divide6/2
  Add2/1 -> Divide3/1
  Mux1/1 -> px/1
  Divide5/1 -> Mux1/1
  Divide3/1 -> Mux1/2

== system dev_switch_ekf/Switching EKF/EKF-DOF=15/corrector/ZMP Calculator/Feet ZMP Calculator L ==
  force : Inport  OutDataType=sfix(16)  OutScaling=2^0
  Enable : EnablePort  StatesWhenEnabling=reset
  Add : Sum  Inputs=--  OutDataType=sfix(16)  OutScaling=2^-10
  Add1 : Sum  Inputs=-+  OutDataType=sfix(16)  OutScaling=2^-10
  Demux : Demux  Outputs=6
  Divide : Product  Inputs=*/  OutDataType=sfix(16)  OutScaling=2^-10
  Divide1 : Product  Inputs=*/  OutDataType=sfix(16)  OutScaling=2^-10
  Gain : Gain  Gain=l_fts  ParameterDataType=sfix(16)  ParameterScaling=2^0  OutDataType=sfix(16)  OutScaling=2^0
  Gain1 : Gain  Gain=l_fts  ParameterDataType=sfix(16)  ParameterScaling=2^0  OutDataType=sfix(16)  OutScaling=2^0
  Mux1 : Mux  Inputs=2
  Terminator1 : Terminator
  FeetZMP* : Outport  OutDataType=sfix(16)  OutScaling=2^0
  wires:
  Demux/6 -> Terminator1/1
  Divide1/1 -> Mux1/2
  Divide/1 -> Mux1/1
  Demux/4 -> Add1/2
  Demux/2 -> Gain1/1
  Demux/3 -> Divide1/2, Divide/2
  Add1/1 -> Divide1/1
  Gain1/1 -> Add1/1
  force/1 -> Demux/1
  Add/1 -> Divide/1
  Demux/5 -> Add/2
  Demux/1 -> Gain/1
  Gain/1 -> Add/1
  Mux1/1 -> FeetZMP*/1

== system dev_switch_ekf/Switching EKF/EKF-DOF=15/corrector/ZMP Calculator/Feet ZMP Calculator R ==
  force : Inport  OutDataType=sfix(16)  OutScaling=2^0
  Enable : EnablePort  StatesWhenEnabling=reset
  Add : Sum  Inputs=--  OutDataType=sfix(16)  OutScaling=2^-10
  Add1 : Sum  Inputs=-+  OutDataType=sfix(16)  OutScaling=2^-10
  Demux : Demux  Outputs=6
  Divide : Product  Inputs=*/  OutDataType=sfix(16)  OutScaling=2^-10
  Divide1 : Product  Inputs=*/  OutDataType=sfix(16)  OutScaling=2^-10
  Gain : Gain  Gain=l_fts  ParameterDataType=sfix(16)  ParameterScaling=2^0  OutDataType=sfix(16)  OutScaling=2^0
  Gain1 : Gain  Gain=l_fts  ParameterDataType=sfix(16)  ParameterScaling=2^0  OutDataType=sfix(16)  OutScaling=2^0
  Mux1 : Mux  Inputs=2
  Terminator1 : Terminator
  FeetZMP* : Outport  OutDataType=sfix(16)  OutScaling=2^0
  wires:
  Demux/6 -> Terminator1/1
  Gain/1 -> Add/1
  Demux/1 -> Gain/1
  Demux/5 -> Add/2
  Add/1 -> Divide/1
  force/1 -> Demux/1
  Gain1/1 -> Add1/1
  Add1/1 -> Divide1/1
  Demux/3 -> Divide/2, Divide1/2
  Demux/2 -> Gain1/1
  Demux/4 -> Add1/2
  Mux1/1 -> FeetZMP*/1
  Divide/1 -> Mux1/1
  Divide1/1 -> Mux1/2

== system dev_switch_ekf/Switching EKF/EKF-DOF=15/corrector/ZMP Calculator/Force Hysteresis ==
  F : Inport
  Compare To Constant : simulink/Logic and Bit Operations/Compare To Constant  SystemSampleTime=-1  relop=<=  const=f0-d  LogicOutDataTypeMode=uint8  ZeroCross=off
  Compare To Constant1 : simulink/Logic and Bit Operations/Compare To Constant  SystemSampleTime=-1  relop=>=  const=f0+d  LogicOutDataTypeMode=uint8  ZeroCross=off
  Constant1 : Constant  OutDataType=sfix(16)  OutScaling=2^0
  Constant2 : Constant  Value=0  OutDataType=sfix(16)  OutScaling=2^0
  Switch : Switch  Threshold=0.5  OutDataType=sfix(16)  OutScaling=2^0
  Switch1 : Switch  Threshold=0.5  OutDataType=sfix(16)  OutScaling=2^0
  Unit Delay : UnitDelay  X0=1  SampleTime=ts
  contact : Outport  OutDataType=sfix(16)  OutScaling=2^0
  wires:
  F/1 -> Compare To Constant1/1, Compare To Constant/1
  Switch/1 -> contact/1, Unit Delay/1
  Unit Delay/1 -> Switch1/3
  Switch1/1 -> Switch/3
  Constant2/1 -> Switch1/1
  Constant1/1 -> Switch/1
  Compare To Constant1/1 -> Switch/2
  Compare To Constant/1 -> Switch1/2

== system dev_switch_ekf/Switching EKF/EKF-DOF=15/corrector/ZMP Calculator/Force Hysteresis1 ==
  F : Inport
  Compare To Constant : simulink/Logic and Bit Operations/Compare To Constant  SystemSampleTime=-1  relop=<=  const=f0-d  LogicOutDataTypeMode=uint8  ZeroCross=off
  Compare To Constant1 : simulink/Logic and Bit Operations/Compare To Constant  SystemSampleTime=-1  relop=>=  const=f0+d  LogicOutDataTypeMode=uint8  ZeroCross=off
  Constant1 : Constant  OutDataType=sfix(16)  OutScaling=2^0
  Constant2 : Constant  Value=0  OutDataType=sfix(16)  OutScaling=2^0
  Switch : Switch  Threshold=0.5  OutDataType=sfix(16)  OutScaling=2^0
  Switch1 : Switch  Threshold=0.5  OutDataType=sfix(16)  OutScaling=2^0
  Unit Delay : UnitDelay  X0=1  SampleTime=ts
  contact : Outport  OutDataType=sfix(16)  OutScaling=2^0
  wires:
  Compare To Constant/1 -> Switch1/2
  Compare To Constant1/1 -> Switch/2
  Constant1/1 -> Switch/1
  Constant2/1 -> Switch1/1
  Switch1/1 -> Switch/3
  Unit Delay/1 -> Switch1/3
  Switch/1 -> Unit Delay/1, contact/1
  F/1 -> Compare To Constant/1, Compare To Constant1/1

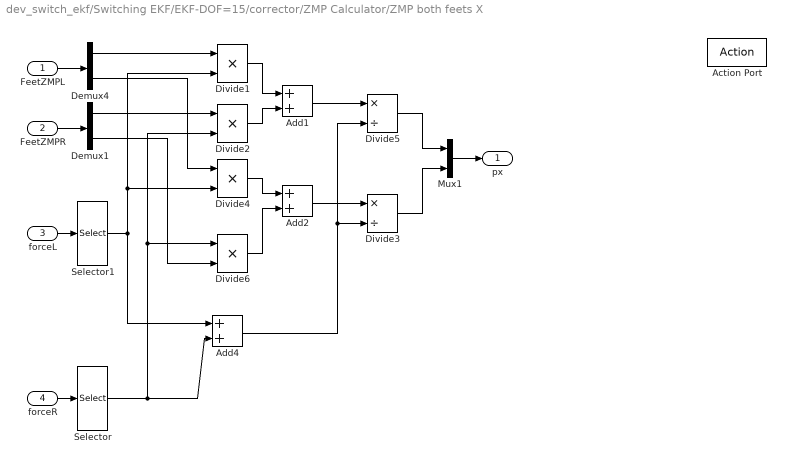
== system dev_switch_ekf/Switching EKF/EKF-DOF=15/corrector/ZMP Calculator/ZMP both feets X ==
  FeetZMPL : Inport  OutDataType=sfix(16)  OutScaling=2^0
  FeetZMPR : Inport  Port=2  OutDataType=sfix(16)  OutScaling=2^0
  forceL : Inport  Port=3  OutDataType=sfix(16)  OutScaling=2^0
  forceR : Inport  Port=4  OutDataType=sfix(16)  OutScaling=2^0
  Action Port : ActionPort  ActionType=then
  Add1 : Sum  OutDataType=sfix(16)  OutScaling=2^-10
  Add2 : Sum  OutDataType=sfix(16)  OutScaling=2^-10
  Add4 : Sum  OutDataType=sfix(16)  OutScaling=2^-10
  Demux1 : Demux  Outputs=2
  Demux4 : Demux  Outputs=2
  Divide{1..2,4,6} (4 alike) : Product  Inputs=**  OutDataType=sfix(16)  OutScaling=2^-10
  Divide3 : Product  Inputs=*/  OutDataType=sfix(16)  OutScaling=2^-10
  Divide5 : Product  Inputs=*/  OutDataType=sfix(16)  OutScaling=2^-10
  Mux1 : Mux  Inputs=2
  Selector : Selector  InputPortWidth=6  IndexOptions=Index vector (dialog)  Indices=[3]  OutputSizes=1
  Selector1 : Selector  InputPortWidth=6  IndexOptions=Index vector (dialog)  Indices=[3]  OutputSizes=1
  px : Outport  OutDataType=sfix(16)  OutScaling=2^0
  wires:
  Divide3/1 -> Mux1/2
  Divide5/1 -> Mux1/1
  Mux1/1 -> px/1
  Add2/1 -> Divide3/1
  Demux1/2 -> Divide6/2
  Demux4/2 -> Divide4/1
  Divide6/1 -> Add2/2
  Divide4/1 -> Add2/1
  Demux4/1 -> Divide1/1
  FeetZMPL/1 -> Demux4/1
  Demux1/1 -> Divide2/1
  FeetZMPR/1 -> Demux1/1
  Add4/1 -> Divide3/2, Divide5/2
  Add1/1 -> Divide5/1
  Divide2/1 -> Add1/2
  Divide1/1 -> Add1/1
  forceL/1 -> Selector1/1
  Selector1/1 -> Divide4/2, Divide1/2, Add4/1
  Selector/1 -> Divide6/1, Divide2/2, Add4/2
  forceR/1 -> Selector/1

== system dev_switch_ekf/Switching EKF/EKF-DOF=9/corrector/ZMP Calculator/Feet ZMP Calculator L ==
  force : Inport  OutDataType=sfix(16)  OutScaling=2^0
  Enable : EnablePort  StatesWhenEnabling=reset
  Add : Sum  Inputs=--  OutDataType=sfix(16)  OutScaling=2^-10
  Add1 : Sum  Inputs=-+  OutDataType=sfix(16)  OutScaling=2^-10
  Demux : Demux  Outputs=6
  Divide : Product  Inputs=*/  OutDataType=sfix(16)  OutScaling=2^-10
  Divide1 : Product  Inputs=*/  OutDataType=sfix(16)  OutScaling=2^-10
  Gain : Gain  Gain=l_fts  ParameterDataType=sfix(16)  ParameterScaling=2^0  OutDataType=sfix(16)  OutScaling=2^0
  Gain1 : Gain  Gain=l_fts  ParameterDataType=sfix(16)  ParameterScaling=2^0  OutDataType=sfix(16)  OutScaling=2^0
  Mux1 : Mux  Inputs=2
  Terminator1 : Terminator
  FeetZMP* : Outport  OutDataType=sfix(16)  OutScaling=2^0
  wires:
  Mux1/1 -> FeetZMP*/1
  Gain/1 -> Add/1
  Demux/1 -> Gain/1
  Demux/5 -> Add/2
  Add/1 -> Divide/1
  force/1 -> Demux/1
  Gain1/1 -> Add1/1
  Add1/1 -> Divide1/1
  Demux/3 -> Divide/2, Divide1/2
  Demux/2 -> Gain1/1
  Demux/4 -> Add1/2
  Divide/1 -> Mux1/1
  Divide1/1 -> Mux1/2
  Demux/6 -> Terminator1/1

== system dev_switch_ekf/Switching EKF/EKF-DOF=9/corrector/ZMP Calculator/Feet ZMP Calculator R ==
  force : Inport  OutDataType=sfix(16)  OutScaling=2^0
  Enable : EnablePort  StatesWhenEnabling=reset
  Add : Sum  Inputs=--  OutDataType=sfix(16)  OutScaling=2^-10
  Add1 : Sum  Inputs=-+  OutDataType=sfix(16)  OutScaling=2^-10
  Demux : Demux  Outputs=6
  Divide : Product  Inputs=*/  OutDataType=sfix(16)  OutScaling=2^-10
  Divide1 : Product  Inputs=*/  OutDataType=sfix(16)  OutScaling=2^-10
  Gain : Gain  Gain=l_fts  ParameterDataType=sfix(16)  ParameterScaling=2^0  OutDataType=sfix(16)  OutScaling=2^0
  Gain1 : Gain  Gain=l_fts  ParameterDataType=sfix(16)  ParameterScaling=2^0  OutDataType=sfix(16)  OutScaling=2^0
  Mux1 : Mux  Inputs=2
  Terminator1 : Terminator
  FeetZMP* : Outport  OutDataType=sfix(16)  OutScaling=2^0
  wires:
  Divide1/1 -> Mux1/2
  Divide/1 -> Mux1/1
  Mux1/1 -> FeetZMP*/1
  Demux/4 -> Add1/2
  Demux/2 -> Gain1/1
  Demux/3 -> Divide1/2, Divide/2
  Add1/1 -> Divide1/1
  Gain1/1 -> Add1/1
  force/1 -> Demux/1
  Add/1 -> Divide/1
  Demux/5 -> Add/2
  Demux/1 -> Gain/1
  Gain/1 -> Add/1
  Demux/6 -> Terminator1/1

== system dev_switch_ekf/Switching EKF/EKF-DOF=9/corrector/ZMP Calculator/Force Hysteresis ==
  F : Inport
  Compare To Constant : simulink/Logic and Bit Operations/Compare To Constant  SystemSampleTime=-1  relop=<=  const=f0-d  LogicOutDataTypeMode=uint8  ZeroCross=off
  Compare To Constant1 : simulink/Logic and Bit Operations/Compare To Constant  SystemSampleTime=-1  relop=>=  const=f0+d  LogicOutDataTypeMode=uint8  ZeroCross=off
  Constant1 : Constant  OutDataType=sfix(16)  OutScaling=2^0
  Constant2 : Constant  Value=0  OutDataType=sfix(16)  OutScaling=2^0
  Switch : Switch  Threshold=0.5  OutDataType=sfix(16)  OutScaling=2^0
  Switch1 : Switch  Threshold=0.5  OutDataType=sfix(16)  OutScaling=2^0
  Unit Delay : UnitDelay  X0=1  SampleTime=ts
  contact : Outport  OutDataType=sfix(16)  OutScaling=2^0
  wires:
  Compare To Constant/1 -> Switch1/2
  Compare To Constant1/1 -> Switch/2
  Constant1/1 -> Switch/1
  Constant2/1 -> Switch1/1
  Switch1/1 -> Switch/3
  Unit Delay/1 -> Switch1/3
  Switch/1 -> Unit Delay/1, contact/1
  F/1 -> Compare To Constant/1, Compare To Constant1/1

== system dev_switch_ekf/Switching EKF/EKF-DOF=9/corrector/ZMP Calculator/Force Hysteresis1 ==
  F : Inport
  Compare To Constant : simulink/Logic and Bit Operations/Compare To Constant  SystemSampleTime=-1  relop=<=  const=f0-d  LogicOutDataTypeMode=uint8  ZeroCross=off
  Compare To Constant1 : simulink/Logic and Bit Operations/Compare To Constant  SystemSampleTime=-1  relop=>=  const=f0+d  LogicOutDataTypeMode=uint8  ZeroCross=off
  Constant1 : Constant  OutDataType=sfix(16)  OutScaling=2^0
  Constant2 : Constant  Value=0  OutDataType=sfix(16)  OutScaling=2^0
  Switch : Switch  Threshold=0.5  OutDataType=sfix(16)  OutScaling=2^0
  Switch1 : Switch  Threshold=0.5  OutDataType=sfix(16)  OutScaling=2^0
  Unit Delay : UnitDelay  X0=1  SampleTime=ts
  contact : Outport  OutDataType=sfix(16)  OutScaling=2^0
  wires:
  F/1 -> Compare To Constant1/1, Compare To Constant/1
  Switch/1 -> contact/1, Unit Delay/1
  Unit Delay/1 -> Switch1/3
  Switch1/1 -> Switch/3
  Constant2/1 -> Switch1/1
  Constant1/1 -> Switch/1
  Compare To Constant1/1 -> Switch/2
  Compare To Constant/1 -> Switch1/2
